simulink model "Inverse_dynamic"  (R2020b)
settings: Solver=FixedStepAuto  StartTime=0.0  StopTime=20  RelTol=1e-3
(part 1 of 4)
settings Model: Creator=Alireza  LastModifiedBy=Asus
settings DataIOCC: ReturnWorkspaceOutputs=off
settings DebuggingCC: ArithmeticOperatorsInVariantConditions=warning
settings SFSimCC: SimUseLocalCustomCode=off  CustomCodeUndefinedFunction=UseInterfaceOnly
settings RTWCC: RTWUseLocalCustomCode=off

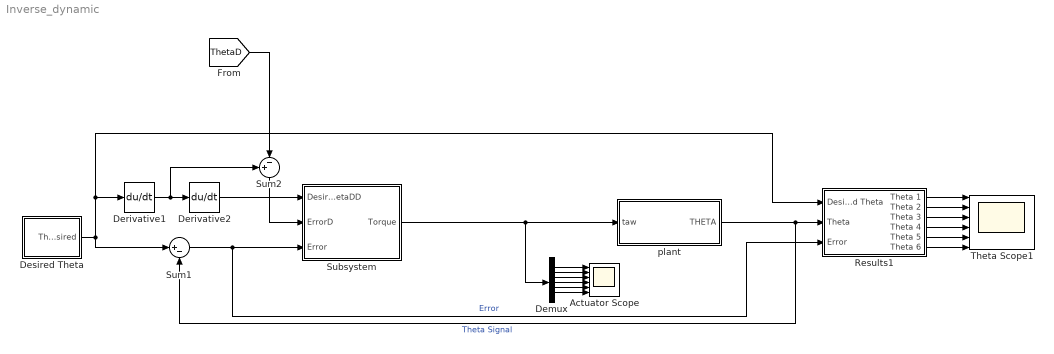
== system Inverse_dynamic ==
  Actuator Scope : Scope  NumInputPorts=6
  Demux : Demux  Outputs=6
  Derivative1 : Derivative
  Derivative2 : Derivative
  Desired Theta : Subsystem
  Results1 : Subsystem
  Subsystem : Subsystem
  Sum1 : Sum  Inputs=|+-
  Sum2 : Sum  Inputs=+-|
  Theta Scope1 : Scope  NumInputPorts=6
  plant : Subsystem
  wires:
  Subsystem/1("Torque ") -> plant/1(taw), Demux/1
  plant/1(THETA) -> Results1/2(Theta), Sum1/2  "Theta Signal"
  Sum1/1 -> Results1/3(Error), Subsystem/3(Error)  "Error"
  Desired Theta/1(Theta Desired) -> Sum1/1, Results1/1(Desired Theta), Derivative1/1
  Demux/1 -> Actuator Scope/1
  Demux/2 -> Actuator Scope/2
  Demux/3 -> Actuator Scope/3
  Demux/4 -> Actuator Scope/4
  Demux/5 -> Actuator Scope/5
  Demux/6 -> Actuator Scope/6
  Derivative2/1 -> Subsystem/1(Desired ThetaDD)
  Sum2/1 -> Subsystem/2(ErrorD)
  Derivative1/1 -> Sum2/1, Derivative2/1
  [ThetaD] -> Sum2/2
  Results1/5(Theta 5) -> Theta Scope1/5
  Results1/4(Theta 4) -> Theta Scope1/4
  Results1/3(Theta 3) -> Theta Scope1/3
  Results1/1(Theta 1) -> Theta Scope1/1
  Results1/2(Theta 2) -> Theta Scope1/2
  Results1/6(Theta 6) -> Theta Scope1/6

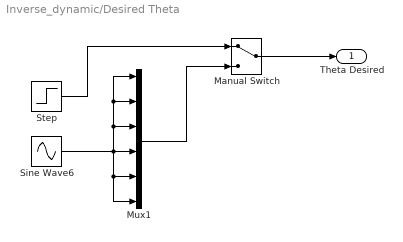
== system Inverse_dynamic/Desired Theta ==
  Manual Switch : ManualSwitch
  Mux1 : Mux  Inputs=6
  Sine Wave6 : Sin  SampleTime=0
  Step : Step  Time=0  Before=[0;0;0;0;0;0];  After=[1;1;1;1;1;1];  SampleTime=0
  Theta Desired : Outport  VectorParamsAs1DForOutWhenUnconnected=off
  wires:
  Sine Wave6/1 -> Mux1/1, Mux1/2, Mux1/3, Mux1/6, Mux1/5, Mux1/4
  Step/1 -> Manual Switch/1
  Manual Switch/1 -> Theta Desired/1
  Mux1/1 -> Manual Switch/2

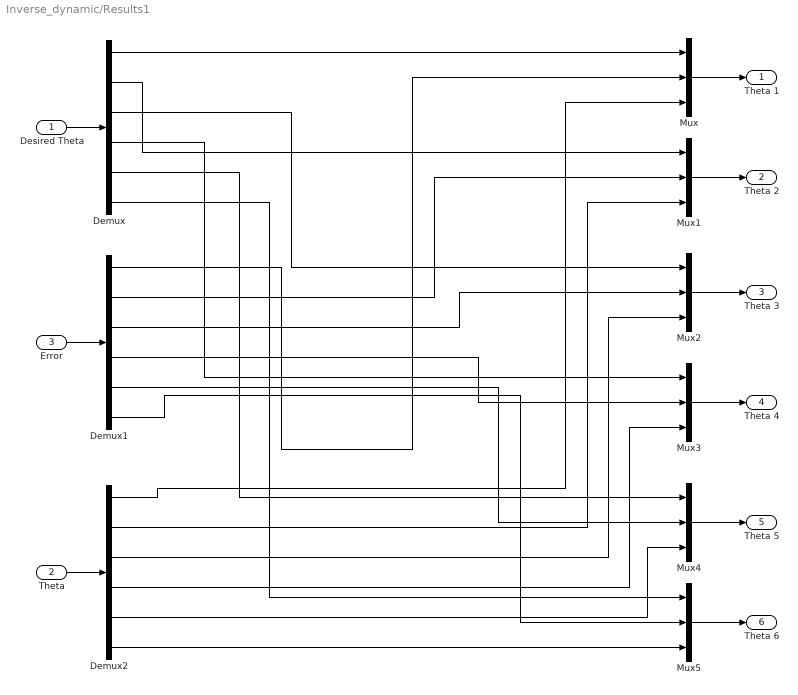
== system Inverse_dynamic/Results1 ==
  Desired Theta : Inport
  Theta : Inport  Port=2
  Error : Inport  Port=3
  Demux : Demux  Outputs=6
  Demux1 : Demux  Outputs=6
  Demux2 : Demux  Outputs=6
  Mux{,1..5} (6 alike) : Mux  Inputs=3
  Theta 1 : Outport  VectorParamsAs1DForOutWhenUnconnected=off
  Theta 2 : Outport  Port=2  VectorParamsAs1DForOutWhenUnconnected=off
  Theta 3 : Outport  Port=3  VectorParamsAs1DForOutWhenUnconnected=off
  Theta 4 : Outport  Port=4  VectorParamsAs1DForOutWhenUnconnected=off
  Theta 5 : Outport  Port=5  VectorParamsAs1DForOutWhenUnconnected=off
  Theta 6 : Outport  Port=6  VectorParamsAs1DForOutWhenUnconnected=off
  wires:
  Desired Theta/1 -> Demux/1
  Error/1 -> Demux1/1
  Theta/1 -> Demux2/1
  Demux/1 -> Mux/1
  Demux/2 -> Mux1/1
  Demux/3 -> Mux2/1
  Demux/4 -> Mux3/1
  Demux/5 -> Mux4/1
  Demux/6 -> Mux5/1
  Demux1/1 -> Mux/2
  Demux1/2 -> Mux1/2
  Demux1/3 -> Mux2/2
  Demux1/4 -> Mux3/2
  Demux1/5 -> Mux4/2
  Demux1/6 -> Mux5/2
  Demux2/1 -> Mux/3
  Demux2/2 -> Mux1/3
  Demux2/3 -> Mux2/3
  Demux2/4 -> Mux3/3
  Demux2/5 -> Mux4/3
  Demux2/6 -> Mux5/3
  Mux/1 -> Theta 1/1
  Mux1/1 -> Theta 2/1
  Mux2/1 -> Theta 3/1
  Mux3/1 -> Theta 4/1
  Mux4/1 -> Theta 5/1
  Mux5/1 -> Theta 6/1

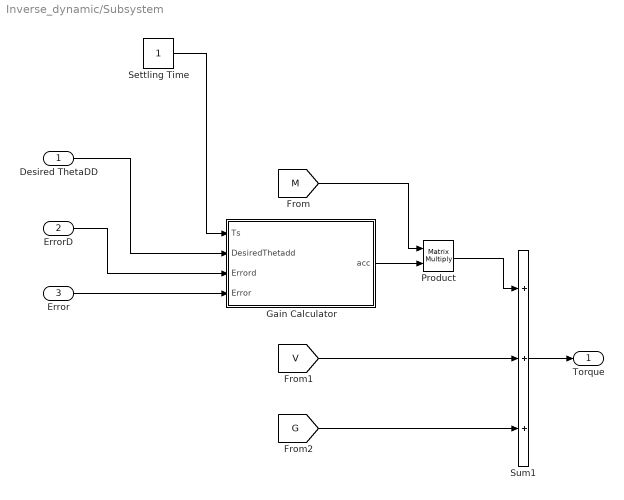
== system Inverse_dynamic/Subsystem ==
  Desired ThetaDD : Inport
  ErrorD : Inport  Port=2
  Error : Inport  Port=3
  Gain Calculator : MATLAB Function  TreatAsAtomicUnit=on
  Product : Product  Multiplication=Matrix(*)
  Settling Time : Constant
  Sum1 : Sum  Inputs=+++
  "Torque " : Outport  VectorParamsAs1DForOutWhenUnconnected=off
  wires:
  [M] -> Product/1
  Gain Calculator/1(acc) -> Product/2
  Product/1 -> Sum1/1
  [V] -> Sum1/2
  [G] -> Sum1/3
  Settling Time/1 -> Gain Calculator/1(Ts)
  ErrorD/1 -> Gain Calculator/3(Errord)
  Error/1 -> Gain Calculator/4(Error)
  Desired ThetaDD/1 -> Gain Calculator/2(DesiredThetadd)
  Sum1/1 -> "Torque "/1

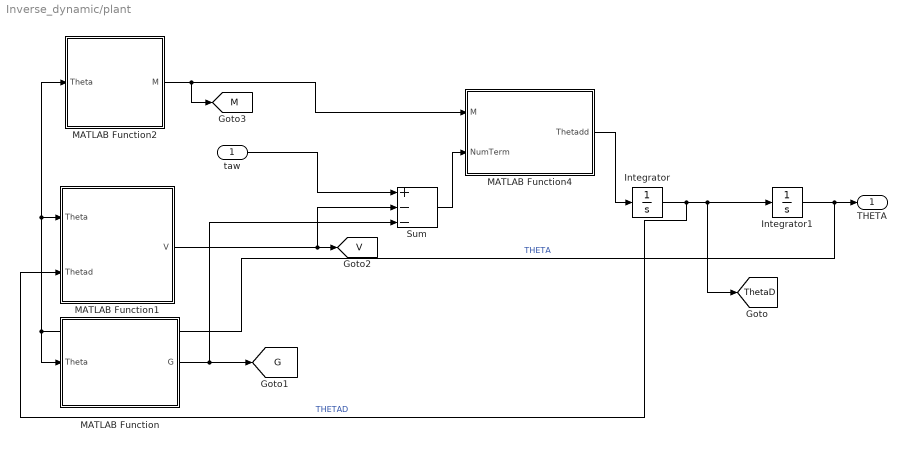
== system Inverse_dynamic/plant ==
  taw : Inport
  Integrator : Integrator  InitialCondition=[0;0;0;0;0;0]
  Integrator1 : Integrator  InitialCondition=[0;0;0;0;0;0]
  MATLAB Function : MATLAB Function  TreatAsAtomicUnit=on
  MATLAB Function1 : MATLAB Function  TreatAsAtomicUnit=on
  MATLAB Function2 : MATLAB Function  TreatAsAtomicUnit=on
  MATLAB Function4 : MATLAB Function  TreatAsAtomicUnit=on
  Sum : Sum  Inputs=+--
  THETA : Outport
  tag scope: G=global, M=global, ThetaD=global, V=global
  wires:
  Integrator/1 -> MATLAB Function1/2(Thetad), [ThetaD], Integrator1/1  "THETAD"
  MATLAB Function4/1(Thetadd) -> Integrator/1
  MATLAB Function1/1(V) -> Sum/2, [V]
  MATLAB Function2/1(M) -> [M], MATLAB Function4/1(M)
  Sum/1 -> MATLAB Function4/2(NumTerm)
  Integrator1/1 -> MATLAB Function1/1(Theta), MATLAB Function2/1(Theta), MATLAB Function/1(Theta), THETA/1  "THETA"
  taw/1 -> Sum/1
  MATLAB Function/1(G) -> Sum/3, [G]
